simulink model "TxSteering_RxMVDR_4x4_HDL_IQ"  (R2021b)
settings: Solver=FixedStepDiscrete  StartTime=0.0  StopTime=stoptime  RelTol=1e-3
PreLoadFcn:
  | model_init
InitFcn:
  | model_init
model workspace (MAT data in the model file):
  socvcb : containers.Map (value not decoded)
values from neighbouring files (symbols this model uses):
  fc = ConverterSampleRate/4    (= 491520000)    [model_init.m]
  FPGAClkRate = DataSampleRate/VectorSamplingFactor    (= 245760000)    [model_init.m]
  movavg_bitshift = nextpow2(sqrt(windowSize))    [model_init.m]
  mvdrPipelineDelay = covMatDelay+movAvgDelay+matrixDivDelay+normResponseDelay    [model_init.m]
  NCO_bits = 14    [model_init.m]
  numArrayElements = 4    [model_init.m]
  S2MM_frame_size = testSrc1.FrameLength*testSrc1.SamplesPerSymbol*3    [model_init.m]
  testSrc1 = struct()    [model_init.m]
  testSrc2 = struct()    [model_init.m]
  windowSize = 4096    [model_init.m]
undefined symbols (not defined in the file or in its folder): j, physconst
libraries: hdlsllib x19, simulink x12, dspsrcs4 x2, embsystolicmatrixops x1, embreciprocals x1, dsphdlsigops x1, commrfcorlib x1
(part 2 of 3)

== system TxSteering_RxMVDR_4x4_HDL_IQ/DUT/Rx Data Capture/Stream FIFO  ==
  dataIn : Inport
  validIn : Inport  Port=2
  readyIn : Inport  Port=3
  Display : Display
  Logical Operator4 : Logic  Operator=NOT  IconShape=distinctive  AllPortsSameDT=off  OutDataTypeStr=boolean
  Logical Operator5 : Logic  IconShape=distinctive  AllPortsSameDT=off  OutDataTypeStr=boolean
  Logical Operator6 : Logic  Operator=NOT  IconShape=distinctive  AllPortsSameDT=off  OutDataTypeStr=boolean
  Logical Operator7 : Logic  IconShape=distinctive  AllPortsSameDT=off  OutDataTypeStr=boolean
  Signal Specification : SignalSpecification  SampleTime=1/FPGAClkRate
  Terminator : Terminator
  hdl_fwft_fifo : Subsystem  mask{FIFO_DEPTH=8192, AFULL_THRESH=4}
      mask prompts: FIFO_DEPTH "FIFO Depth"; AFULL_THRESH "Almost Full Threshold"
      mask init:
      | FIFO_CNT_BITS=ceil(log2(FIFO_DEPTH+1+3));
  dataOut : Outport  VectorParamsAs1DForOutWhenUnconnected=off
  ValidOut : Outport  Port=2  VectorParamsAs1DForOutWhenUnconnected=off
  readyOut : Outport  Port=3  VectorParamsAs1DForOutWhenUnconnected=off
  wires:
  Logical Operator4/1 -> Logical Operator5/2
  Logical Operator7/1 -> hdl_fwft_fifo/2(push)
  readyIn/1 -> Logical Operator5/1
  validIn/1 -> Logical Operator7/2
  hdl_fwft_fifo/2(empty) -> Logical Operator4/1
  hdl_fwft_fifo/3(num) -> Display/1
  dataIn/1 -> Signal Specification/1
  hdl_fwft_fifo/1(data_o) -> dataOut/1
  Logical Operator5/1 -> hdl_fwft_fifo/3(rd_ack), ValidOut/1
  Signal Specification/1 -> hdl_fwft_fifo/1(data_i)
  hdl_fwft_fifo/4(full) -> Terminator/1
  Logical Operator6/1 -> readyOut/1, Logical Operator7/1
  hdl_fwft_fifo/5(afull) -> Logical Operator6/1

== system TxSteering_RxMVDR_4x4_HDL_IQ/DUT/Rx Input Preparation/Apply Calibration Coefficients ==
  dataIn : Inport
  validIn : Inport  Port=2
  coeffIn : Inport  Port=3
  Data Type Duplicate : DataTypeDuplicate
  Data Type Conversion : DataTypeConversion
  Data Type Conversion1 : DataTypeConversion  OutDataTypeStr=input_dt  ConvertRealWorld=Stored Integer (SI)
  For Each Subsystem : Subsystem  TreatAsAtomicUnit=on
  Reshape : Reshape
  Reshape1 : Reshape  OutputDimensionality=Row vector (2-D)
  Reshape2 : Reshape
  Reshape3 : Reshape
  Selector : Selector  InputPortWidth=4  IndexOptions=Index vector (dialog)  Indices=1  OutputSizes=1
  dataOut : Outport
  validOut : Outport  Port=2
  wires:
  Data Type Conversion/1 -> Reshape1/1, Data Type Duplicate/2
  Reshape3/1 -> For Each Subsystem/3(coeffIn)
  Reshape2/1 -> For Each Subsystem/1(dataIn), Data Type Duplicate/1
  Reshape1/1 -> dataOut/1
  Reshape/1 -> Selector/1
  Selector/1 -> validOut/1
  For Each Subsystem/1(dataOut) -> Data Type Conversion/1
  For Each Subsystem/2(validOut) -> Reshape/1
  validIn/1 -> For Each Subsystem/2(validIn)
  dataIn/1 -> Data Type Conversion1/1
  coeffIn/1 -> Reshape3/1
  Data Type Conversion1/1 -> Reshape2/1

== system TxSteering_RxMVDR_4x4_HDL_IQ/DUT/Rx Input Preparation/From Data Bus ==
  bus : Inport
  Bus Selector : BusSelector  OutputSignals=data,valid
  data : Outport  VectorParamsAs1DForOutWhenUnconnected=off
  valid : Outport  Port=2  VectorParamsAs1DForOutWhenUnconnected=off
  wires:
  Bus Selector/2 -> valid/1  "<valid>"
  Bus Selector/1 -> data/1  "<data>"
  bus/1 -> Bus Selector/1

== system TxSteering_RxMVDR_4x4_HDL_IQ/DUT/Rx Input Preparation/To Data Bus ==
  data : Inport
  valid : Inport  Port=2
  Bus Creator : BusCreator  Inputs=2
  bus : Outport  VectorParamsAs1DForOutWhenUnconnected=off
  wires:
  valid/1 -> Bus Creator/2  "valid"
  data/1 -> Bus Creator/1  "data"
  Bus Creator/1 -> bus/1

== system TxSteering_RxMVDR_4x4_HDL_IQ/DUT/To DAC Interface/From Data Bus ==
  bus : Inport
  Bus Selector : BusSelector  OutputSignals=data,valid
  data : Outport  VectorParamsAs1DForOutWhenUnconnected=off
  valid : Outport  Port=2  VectorParamsAs1DForOutWhenUnconnected=off
  wires:
  Bus Selector/2 -> valid/1  "<valid>"
  Bus Selector/1 -> data/1  "<data>"
  bus/1 -> Bus Selector/1

== system TxSteering_RxMVDR_4x4_HDL_IQ/DUT/Tx Signal Generation/Calibration NCO ==
  inc : Inport
  Constant : Constant  Value=true  SampleTime=-1
  Data Type Conversion : DataTypeConversion  OutDataTypeStr=input_dt
  Mux : Mux
  NCO HDL Optimized : dsphdlsigops/NCO HDL Optimized  PhaseIncrementSource=Input port  PhaseIncrement=100  PhaseOffsetSource=Property  PhaseOffset=0  DitherSource=Property  NumDitherBits=4  SamplesPerFrame=1  LUTCompress=off  ResetAction=off  Waveform=Complex exponential  PhasePort=off  SimulateUsing=Code generation  AccumulatorWL=NCO_bits  PhaseQuantization=on  NumQuantizerAccumulatorBits=12  OutputDataType=Binary point scaling  OutputWL=NCO_bits  OutputFL=NCO_bits-1
      settings: SourceProductName=DSP System Toolbox HDL Support
  dataOut : Outport
  validOut : Outport  Port=2
  wires:
  inc/1 -> NCO HDL Optimized/1
  NCO HDL Optimized/2 -> validOut/1
  Constant/1 -> NCO HDL Optimized/2
  NCO HDL Optimized/1 -> Data Type Conversion/1
  Data Type Conversion/1 -> Mux/1, Mux/2, Mux/3, Mux/4
  Mux/1 -> dataOut/1

== system TxSteering_RxMVDR_4x4_HDL_IQ/DUT/Tx Signal Generation/Combine Channels ==
  dataIn : Inport
  validIn : Inport  Port=2
  Add : Sum
  Bit Shift : hdlsllib/Logic and Bit Operations/Bit Shift  mode=Shift Right Arithmetic  N=1
  Data Type Conversion : DataTypeConversion  OutDataTypeStr=int16
  Data Type Conversion1 : DataTypeConversion  OutDataTypeStr=input_dt  ConvertRealWorld=Stored Integer (SI)
  Delay{,1..4} (5 alike) : Delay  DelayLength=1
  Selector : Selector  InputPortWidth=2  IndexOptions=Index vector (dialog)  Indices=1  OutputSizes=1
  Selector1 : Selector  InputPortWidth=8  IndexOptions=Index vector (dialog)  Indices=1:4  OutputSizes=1
  Selector2 : Selector  InputPortWidth=8  IndexOptions=Index vector (dialog)  Indices=5:8  OutputSizes=1
  dataOut : Outport
  validOut : Outport  Port=2
  wires:
  Bit Shift/1 -> Data Type Conversion/1
  dataIn/1 -> Selector2/1, Selector1/1
  validIn/1 -> Selector/1
  Selector/1 -> Delay3/1
  Selector2/1 -> Delay1/1
  Selector1/1 -> Delay/1
  Delay/1 -> Add/1
  Delay1/1 -> Add/2
  Delay2/1 -> Bit Shift/1
  Add/1 -> Delay2/1
  Delay3/1 -> Delay4/1
  Delay4/1 -> validOut/1
  Data Type Conversion/1 -> Data Type Conversion1/1
  Data Type Conversion1/1 -> dataOut/1

== system TxSteering_RxMVDR_4x4_HDL_IQ/DUT/Tx Signal Generation/Generate Steering Channels ==
  dataIn : Inport  Partition=on  PartitionDimension=1  PartitionWidth=1  PartitionOffset=0
  validIn : Inport  Port=2
  gain : Inport  Port=3  Partition=on  PartitionDimension=1  PartitionWidth=1  PartitionOffset=0
  steeringCoeffs : Inport  Port=4  Partition=on  PartitionDimension=1  PartitionWidth=4  PartitionOffset=0
  Apply Gain : Subsystem
  Apply Steering Coefficients : Subsystem  TreatAsAtomicUnit=on
  Data Type Conversion : DataTypeConversion  OutDataTypeStr=fixdt(1,16,0)
  For Each : ForEach  DisableCoverage=on
  Selector : Selector  InputPortWidth=4  IndexOptions=Index vector (dialog)  Indices=1  OutputSizes=1
  dataOut : Outport  ConcatenationDimension=1
  validOut : Outport  Port=2  ConcatenationDimension=1
  wires:
  Data Type Conversion/1 -> dataOut/1
  Selector/1 -> validOut/1
  steeringCoeffs/1 -> Apply Steering Coefficients/3(coeffIn)
  Apply Steering Coefficients/1(dataOut) -> Data Type Conversion/1
  Apply Steering Coefficients/2(validOut) -> Selector/1
  Apply Gain/1(dataOut) -> Apply Steering Coefficients/1(dataIn)
  gain/1 -> Apply Gain/3(gain)
  Apply Gain/2(validOut) -> Apply Steering Coefficients/2(validIn)
  dataIn/1 -> Apply Gain/1(dataIn)
  validIn/1 -> Apply Gain/2(validIn)

== system TxSteering_RxMVDR_4x4_HDL_IQ/DUT/Tx Signal Generation/To Data Bus ==
  data : Inport
  valid : Inport  Port=2
  Bus Creator : BusCreator  Inputs=2
  bus : Outport  VectorParamsAs1DForOutWhenUnconnected=off
  wires:
  Bus Creator/1 -> bus/1
  data/1 -> Bus Creator/1  "data"
  valid/1 -> Bus Creator/2  "valid"

== system TxSteering_RxMVDR_4x4_HDL_IQ/DUT/Tx Signal Generation/To Data Bus1 ==
  data : Inport
  valid : Inport  Port=2
  Bus Creator : BusCreator  Inputs=2
  bus : Outport  VectorParamsAs1DForOutWhenUnconnected=off
  wires:
  valid/1 -> Bus Creator/2  "valid"
  data/1 -> Bus Creator/1  "data"
  Bus Creator/1 -> bus/1

== system TxSteering_RxMVDR_4x4_HDL_IQ/DUT/Tx Signal Generation/Tx Source LUT ==
  Constant : Constant  Value=true  SampleTime=-1
  Delay : Delay  DelayLength=1
  HDL Counter : hdlsllib/Sources/HDL Counter  CountType=Count limited  CountInit=0  CountStep=1  CountMax=length(testSrc1.Data)-1  CountFromType=Initial value  CountFrom=0  CountResetPort=off  CountLoadPort=off  CountEnbPort=off  CountDirPort=off  CountHitOutputPort=off  CountDataType=Unsigned  CountWordLen=nextpow2(length(testSrc1.Data))  CountFracLen=0  CountSampTime=1/FPGAClkRate
  HDL Counter1 : hdlsllib/Sources/HDL Counter  CountType=Count limited  CountInit=0  CountStep=1  CountMax=length(testSrc2.Data)-1  CountFromType=Initial value  CountFrom=0  CountResetPort=off  CountLoadPort=off  CountEnbPort=off  CountDirPort=off  CountHitOutputPort=off  CountDataType=Unsigned  CountWordLen=nextpow2(length(testSrc2.Data))  CountFracLen=0  CountSampTime=1/FPGAClkRate
  HW Delay : UnitDelay  SampleTime=-1  HasFrameUpgradeWarning=on
  HW Delay1 : UnitDelay  SampleTime=-1  HasFrameUpgradeWarning=on
  Mux : Mux  Inputs=2
  Source 1 LUT : LookupNDDirect  NumberOfTableDimensions=1  Table=testSrc1.Data  DiagnosticForOutOfRangeInput=Error  TableDataTypeStr=fixdt(1,16,15)
  Source 2 LUT : LookupNDDirect  NumberOfTableDimensions=1  Table=testSrc2.Data  DiagnosticForOutOfRangeInput=Error  TableDataTypeStr=fixdt(1,16,15)
  dataOut : Outport
  validOut : Outport  Port=2
  wires:
  Source 1 LUT/1 -> HW Delay/1
  HDL Counter/1 -> Source 1 LUT/1
  Source 2 LUT/1 -> HW Delay1/1
  HW Delay/1 -> Mux/1
  HW Delay1/1 -> Mux/2
  Mux/1 -> dataOut/1
  Constant/1 -> Delay/1
  Delay/1 -> validOut/1
  HDL Counter1/1 -> Source 2 LUT/1

== system TxSteering_RxMVDR_4x4_HDL_IQ/S2MM DMA Plant/Unpack to uint32/Enabled Subsystem ==
  dataIn : Inport
  Enable : EnablePort
  Extract Bits : simulink/Logic and Bit Operations/Extract Bits  bitsToExtract=Range of bits  numBits=8  bitIdxRange=[0 31]  outScalingMode=Treat bit field as an integer
  Extract Bits1 : simulink/Logic and Bit Operations/Extract Bits  bitsToExtract=Range of bits  numBits=8  bitIdxRange=[32 63]  outScalingMode=Treat bit field as an integer
  Extract Bits2 : simulink/Logic and Bit Operations/Extract Bits  bitsToExtract=Range of bits  numBits=8  bitIdxRange=[64 95]  outScalingMode=Treat bit field as an integer
  Extract Bits3 : simulink/Logic and Bit Operations/Extract Bits  bitsToExtract=Range of bits  numBits=8  bitIdxRange=[96 127]  outScalingMode=Treat bit field as an integer
  Matrix Concatenate : Concatenate  NumInputs=4  Mode=Multidimensional array
  Reshape : Reshape  OutputDimensionality=Row vector (2-D)
  Reshape1 : Reshape
  dataOut : Outport
  wires:
  dataIn/1 -> Reshape/1
  Extract Bits/1 -> Matrix Concatenate/1
  Extract Bits3/1 -> Matrix Concatenate/4
  Extract Bits2/1 -> Matrix Concatenate/3
  Extract Bits1/1 -> Matrix Concatenate/2
  Reshape/1 -> Extract Bits/1, Extract Bits1/1, Extract Bits2/1, Extract Bits3/1
  Matrix Concatenate/1 -> Reshape1/1
  Reshape1/1 -> dataOut/1

== system TxSteering_RxMVDR_4x4_HDL_IQ/DUT/Rx Beamforming/Input Gate/From Data Bus ==
  bus : Inport
  Bus Selector : BusSelector  OutputSignals=data,valid
  data : Outport  VectorParamsAs1DForOutWhenUnconnected=off
  valid : Outport  Port=2  VectorParamsAs1DForOutWhenUnconnected=off
  wires:
  Bus Selector/2 -> valid/1  "<valid>"
  Bus Selector/1 -> data/1  "<data>"
  bus/1 -> Bus Selector/1

== system TxSteering_RxMVDR_4x4_HDL_IQ/DUT/Rx Beamforming/Input Gate/To Data Bus ==
  data : Inport
  valid : Inport  Port=2
  Bus Creator : BusCreator  Inputs=2
  bus : Outport  VectorParamsAs1DForOutWhenUnconnected=off
  wires:
  valid/1 -> Bus Creator/2  "valid"
  data/1 -> Bus Creator/1  "data"
  Bus Creator/1 -> bus/1

== system TxSteering_RxMVDR_4x4_HDL_IQ/DUT/Rx Beamforming/Input Gate/To Data Bus1 ==
  data : Inport
  valid : Inport  Port=2
  Bus Creator : BusCreator  Inputs=2
  bus : Outport  VectorParamsAs1DForOutWhenUnconnected=off
  wires:
  Bus Creator/1 -> bus/1
  data/1 -> Bus Creator/1  "data"
  valid/1 -> Bus Creator/2  "valid"

== system TxSteering_RxMVDR_4x4_HDL_IQ/DUT/Rx Beamforming/MVDR/Compute Weight Vector ==
  covarianceMatrix : Inport
  validIn : Inport  Port=2
  steeringVector : Inport  Port=3
  Complex Partial-Systolic Matrix Solve Using QR Decomposition : embsystolicmatrixops/Complex Partial-Systolic Matrix Solve Using QR Decomposition  m=4  n=4  p=1  regularizationParameter=0  OutputType=fixdt(1,32,15)
      settings: SourceProductBaseCode=SL
  Constant : Constant  Value=false  SampleTime=-1
  Data Type Conversion1 : DataTypeConversion  OutDataTypeStr=matrixdivin_dt
  Data Type Conversion2 : DataTypeConversion  OutDataTypeStr=matrixdivin_dt
  Data Type Conversion4 : DataTypeConversion  OutDataTypeStr=matrixdivout_dt
  Deserialize Output Data : Subsystem
  Reshape1 : Reshape  OutputDimensionality=Column vector (2-D)  OutputDimensions=[4,4]
  Serialize Input Data : Subsystem
  w : Outport
  validOut : Outport  Port=2
  wires:
  covarianceMatrix/1 -> Data Type Conversion1/1
  steeringVector/1 -> Data Type Conversion2/1
  Data Type Conversion2/1 -> Reshape1/1
  validIn/1 -> Serialize Input Data/3(validIn)
  Constant/1 -> Complex Partial-Systolic Matrix Solve Using QR Decomposition/4
  Serialize Input Data/3(validOut) -> Complex Partial-Systolic Matrix Solve Using QR Decomposition/3  "validIn"
  Complex Partial-Systolic Matrix Solve Using QR Decomposition/3 -> Serialize Input Data/4(readyIn)
  Serialize Input Data/1(AOut) -> Complex Partial-Systolic Matrix Solve Using QR Decomposition/1
  Reshape1/1 -> Serialize Input Data/2(BIn)
  Complex Partial-Systolic Matrix Solve Using QR Decomposition/1 -> Data Type Conversion4/1
  Data Type Conversion4/1 -> Deserialize Output Data/1(dataIn)
  Complex Partial-Systolic Matrix Solve Using QR Decomposition/2 -> Deserialize Output Data/2(validIn)
  Deserialize Output Data/1(dataOut) -> w/1
  Deserialize Output Data/2(validOut) -> validOut/1
  Serialize Input Data/2(BOut) -> Complex Partial-Systolic Matrix Solve Using QR Decomposition/2
  Data Type Conversion1/1 -> Serialize Input Data/1(AIn)

== system TxSteering_RxMVDR_4x4_HDL_IQ/DUT/Rx Beamforming/MVDR/Form Beam ==
  Bus Element In : Inport  PortName=dataBusIn  Element=data
  Bus Element In1 : Inport  PortName=dataBusIn  Element=valid
  w : Inport  Port=2
  Data Type Conversion : DataTypeConversion  OutDataTypeStr=output_dt
  Delay1 : Delay  DelayLength=6
  Delay2 : Delay
  Delay3 : Delay  DelayLength=mvdrPipelineDelay
  Delay5 : Delay  DelayLength=mvdrPipelineDelay
  Math Function2 : Math  Operator=conj  SaturateOnIntegerOverflow=on
  Parallel Complex Multiply : Subsystem  TreatAsAtomicUnit=on
  Reshape : Reshape
  Reshape1 : Reshape
  Rx Beam - Spectrum : SpectrumAnalyzer
  Tree Sum : Subsystem
  Bus Element Out : Outport  PortName=dataBusOut  Element=data
  Out Bus Element : Outport  PortName=dataBusOut  Element=valid
  wires:
  Bus Element In/1 -> Delay5/1
  Parallel Complex Multiply/1(z) -> Tree Sum/1(In1)
  Tree Sum/1(Out1) -> Data Type Conversion/1
  Math Function2/1 -> Reshape/1
  w/1 -> Math Function2/1
  Reshape/1 -> Parallel Complex Multiply/2(z2)
  Reshape1/1 -> Parallel Complex Multiply/1(z1)
  Data Type Conversion/1 -> Rx Beam - Spectrum/1, Bus Element Out/1
  Delay2/1 -> Out Bus Element/1
  Delay1/1 -> Delay2/1
  Bus Element In1/1 -> Delay3/1
  Delay5/1 -> Reshape1/1
  Delay3/1 -> Delay1/1

== system TxSteering_RxMVDR_4x4_HDL_IQ/DUT/Rx Beamforming/MVDR/Form Covariance Matrix ==
  Bus Element In : Inport  PortName=dataBusIn  Element=data
  Bus Element In1 : Inport  PortName=dataBusIn  Element=valid
  Conj : Math  Operator=conj
  Data Type Conversion : DataTypeConversion  OutDataTypeStr=covmat_dt
  Data Type Conversion1 : DataTypeConversion  OutDataTypeStr=adc_dt
  Delay : Delay  DelayLength=6
  Matrix Multiply Partitioned : Subsystem  TreatAsAtomicUnit=on
  Reshape : Reshape
  dataOut : Outport
  validOut : Outport  Port=2
  wires:
  Bus Element In1/1 -> Delay/1
  Bus Element In/1 -> Data Type Conversion1/1
  Reshape/1 -> Conj/1, Matrix Multiply Partitioned/1(x)  "x"
  Matrix Multiply Partitioned/1(C) -> Data Type Conversion/1  "x * x'"
  Delay/1 -> validOut/1
  Conj/1 -> Matrix Multiply Partitioned/2(x_conj)
  Data Type Conversion1/1 -> Reshape/1
  Data Type Conversion/1 -> dataOut/1

== system TxSteering_RxMVDR_4x4_HDL_IQ/DUT/Rx Beamforming/MVDR/Moving Average ==
  note: Shift replaces gain by 1/sqrt(windowSize)
  dataIn : Inport
  validIn : Inport  Port=2
  Add : Sum  Inputs=++-  AccumDataTypeStr=movavg_accum_dt  OutDataTypeStr=Inherit: Same as accumulator
  Bit Shift : hdlsllib/Logic and Bit Operations/Bit Shift  mode=Shift Right Arithmetic  N=movavg_bitshift
  Data Type Conversion : DataTypeConversion  OutDataTypeStr=movavg_out_dt
  Delay : Delay  DelayLength=windowSize
  Delay{1..5} (5 alike) : Delay  DelayLength=1
  Reshape : Reshape  OutputDimensionality=Customize  OutputDimensions=[4,4]
  Reshape1 : Reshape  OutputDimensions=[4,4]
  Wait for Running Sum Init : Subsystem
  dataOut : Outport
  validOut : Outport  Port=2
  wires:
  Bit Shift/1 -> Data Type Conversion/1
  Delay1/1 -> Bit Shift/1, Add/1
  Delay/1 -> Add/3
  Add/1 -> Delay1/1
  dataIn/1 -> Delay2/1
  validIn/1 -> Delay3/1
  Delay2/1 -> Reshape1/1
  Delay4/1 -> dataOut/1
  Delay5/1 -> validOut/1
  Delay3/1 -> Wait for Running Sum Init/1(In1)
  Wait for Running Sum Init/1(Out1) -> Delay5/1
  Data Type Conversion/1 -> Reshape/1
  Reshape/1 -> Delay4/1
  Reshape1/1 -> Delay/1, Add/2

== system TxSteering_RxMVDR_4x4_HDL_IQ/DUT/Rx Beamforming/MVDR/Normalize Response ==
  note: This subsystem scales the weight vector to ensure unit gain in the target direction.
  wIn : Inport
  validIn : Inport  Port=2
  steeringVector : Inport  Port=3
  MVDR Weight Update : Subsystem
  Unit Delay Enabled Synchronous : hdlsllib/Discrete/Unit Delay Enabled Synchronous  InitialCondition=0.0  SampleTime=-1
      settings: SourceProductBaseCode=SL
  wOut : Outport
  wires:
  steeringVector/1 -> MVDR Weight Update/1(Steering Vector)
  wIn/1 -> MVDR Weight Update/2(x)
  MVDR Weight Update/1(w) -> Unit Delay Enabled Synchronous/1
  MVDR Weight Update/2(validOut) -> Unit Delay Enabled Synchronous/2
  Unit Delay Enabled Synchronous/1 -> wOut/1
  validIn/1 -> MVDR Weight Update/3(validIn)

== system TxSteering_RxMVDR_4x4_HDL_IQ/DUT/Rx Beamforming/Output Selector/RepackageInput ==
  In1 : Inport
  Bus Creator : BusCreator  Inputs=2
  Bus Selector : BusSelector  OutputSignals=data,valid
  Pack Complex Vector : Subsystem  mask(Pack Complex Vector){}
      mask help:
      | Convert complex vector to packed word.
      |
      | Real and imaginary components are interleaved, with real component starting in LSB position.
      |
      | The first vector element is placed in the LSB, and the last vector element is placed in the MSB.
      mask Display: fprintf('Pack\nComplex\nVector');
  Out1 : Outport
  wires:
  In1/1 -> Bus Selector/1
  Bus Creator/1 -> Out1/1
  Bus Selector/2 -> Bus Creator/2  "<valid>"
  Bus Selector/1 -> Pack Complex Vector/1(u)  "<data>"
  Pack Complex Vector/1(y) -> Bus Creator/1  "data"

== system TxSteering_RxMVDR_4x4_HDL_IQ/DUT/Rx Beamforming/Output Selector/RepackageMVDR ==
  In3 : Inport
  Bus Creator : BusCreator  Inputs=2
  Bus Selector : BusSelector  OutputSignals=data,valid
  Data Type Conversion1 : DataTypeConversion  OutDataTypeStr=fixdt(0,128,0)
  Pack Complex : Subsystem  mask(Pack Complex){dummy=0}
      mask help:
      | Convert complex value to packed word.
      |
      | Real component goes to lower bits; imaginary component goes to upper bits.
      mask Display: fprintf('Pack\nComplex');
  Out1 : Outport
  wires:
  Pack Complex/1(Out1) -> Data Type Conversion1/1
  Data Type Conversion1/1 -> Bus Creator/1  "data"
  Bus Selector/2 -> Bus Creator/2  "<valid>"
  In3/1 -> Bus Selector/1
  Bus Creator/1 -> Out1/1
  Bus Selector/1 -> Pack Complex/1(In1)  "<data>"

== system TxSteering_RxMVDR_4x4_HDL_IQ/DUT/Rx Data Capture/CaptureTriggerControl/AXI4-Lite Initial Value ==
  In1 : Inport
  Compare To Zero : simulink/Logic and Bit Operations/Compare To Zero  relop=~=  OutDataTypeStr=boolean
  Logical Operator : Logic  Operator=OR  IconShape=distinctive  AllPortsSameDT=off  OutDataTypeStr=boolean
  Set_Latch : Subsystem
  Unit Delay Enabled Synchronous : hdlsllib/Discrete/Unit Delay Enabled Synchronous  InitialCondition=x0  SampleTime=-1
      settings: SourceProductBaseCode=SL
  Out1 : Outport  VectorParamsAs1DForOutWhenUnconnected=off
  wires:
  In1/1 -> Unit Delay Enabled Synchronous/1, Compare To Zero/1
  Logical Operator/1 -> Unit Delay Enabled Synchronous/2
  Compare To Zero/1 -> Logical Operator/1, Set_Latch/1(S)
  Set_Latch/1(Q) -> Logical Operator/2
  Unit Delay Enabled Synchronous/1 -> Out1/1

== system TxSteering_RxMVDR_4x4_HDL_IQ/DUT/Rx Data Capture/CaptureTriggerControl/AutoTrigger ==
  MaxCount : Inport
  En : Inport  Port=2
  DataPushFrequency : hdlsllib/Sources/HDL Counter  CountType=Free running  CountInit=0  CountStep=1  CountMax=25  CountFromType=Initial value  CountFrom=0  CountResetPort=on  CountLoadPort=off  CountEnbPort=on  CountDirPort=off  CountHitOutputPort=off  CountDataType=Unsigned  CountWordLen=32  CountFracLen=0  CountSampTime=1
  Relational Operator : RelationalOperator  Operator===  OutDataTypeStr=boolean  RndMeth=Simplest
  Trig : Outport  VectorParamsAs1DForOutWhenUnconnected=off
  wires:
  DataPushFrequency/1 -> Relational Operator/2
  Relational Operator/1 -> Trig/1, DataPushFrequency/1
  En/1 -> DataPushFrequency/2
  MaxCount/1 -> Relational Operator/1

== system TxSteering_RxMVDR_4x4_HDL_IQ/DUT/Rx Data Capture/FIFOControl/HandleDefaultValue ==
  In1 : Inport
  Compare To Zero1 : simulink/Logic and Bit Operations/Compare To Zero  relop=~=  OutDataTypeStr=boolean
  Constant : Constant  Value=1024  OutDataTypeStr=uint32  SampleTime=-1
  Switch : Switch  Criteria=u2 ~= 0
  Out1 : Outport
  wires:
  Compare To Zero1/1 -> Switch/2
  Constant/1 -> Switch/3
  Switch/1 -> Out1/1
  In1/1 -> Compare To Zero1/1, Switch/1

== system TxSteering_RxMVDR_4x4_HDL_IQ/DUT/Rx Data Capture/FIFOControl/sr_latch ==
  S : Inport
  R : Inport  Port=2
  Logical Operator1 : Logic  IconShape=distinctive  AllPortsSameDT=off  OutDataTypeStr=boolean
  Logical Operator2 : Logic  Operator=NOT  IconShape=distinctive  AllPortsSameDT=off  OutDataTypeStr=boolean
  Logical Operator9 : Logic  Operator=OR  IconShape=distinctive  AllPortsSameDT=off  OutDataTypeStr=boolean
  Unit Delay1 : UnitDelay  SampleTime=-1  HasFrameUpgradeWarning=on
  Q : Outport  VectorParamsAs1DForOutWhenUnconnected=off
  wires:
  S/1 -> Logical Operator9/1
  R/1 -> Logical Operator2/1
  Logical Operator2/1 -> Logical Operator1/1
  Unit Delay1/1 -> Logical Operator1/2, Q/1
  Logical Operator9/1 -> Unit Delay1/1
  Logical Operator1/1 -> Logical Operator9/2

== system TxSteering_RxMVDR_4x4_HDL_IQ/DUT/Rx Data Capture/Stream FIFO /hdl_fwft_fifo ==
  data_i : Inport
  push : Inport  Port=2
  rd_ack : Inport  Port=3
  Compare To Constant : simulink/Logic and Bit Operations/Compare To Constant  relop=>=  const=FIFO_DEPTH-AFULL_THRESH  OutDataTypeStr=boolean
  HDL FIFO : hdlsllib/HDL RAMs/HDL FIFO  fifo_size=FIFO_DEPTH  mode=FWFT  ratio=1  push_msg=Error  pop_msg=Ignore  show_empty=on  show_full=on  show_num=on  LabelModeActiveChoice_Mode=FWFT
      settings: SourceProductBaseCode=SL
  Logical Operator1 : Logic  Operator=NOT  IconShape=distinctive  AllPortsSameDT=off  OutDataTypeStr=boolean
  Logical Operator2 : Logic  IconShape=distinctive  AllPortsSameDT=off  OutDataTypeStr=boolean
  data_o : Outport  VectorParamsAs1DForOutWhenUnconnected=off
  empty : Outport  Port=2  VectorParamsAs1DForOutWhenUnconnected=off
  num : Outport  Port=3  VectorParamsAs1DForOutWhenUnconnected=off
  full : Outport  Port=4  VectorParamsAs1DForOutWhenUnconnected=off
  afull : Outport  Port=5  VectorParamsAs1DForOutWhenUnconnected=off
  wires:
  Compare To Constant/1 -> afull/1
  data_i/1 -> HDL FIFO/1
  push/1 -> Logical Operator2/1
  Logical Operator2/1 -> HDL FIFO/2
  Logical Operator1/1 -> Logical Operator2/2
  HDL FIFO/3 -> Logical Operator1/1, full/1
  HDL FIFO/4 -> Compare To Constant/1, num/1
  HDL FIFO/2 -> empty/1
  HDL FIFO/1 -> data_o/1
  rd_ack/1 -> HDL FIFO/3

== system TxSteering_RxMVDR_4x4_HDL_IQ/DUT/Rx Input Preparation/Apply Calibration Coefficients/For Each Subsystem ==
  dataIn : Inport  Partition=on  PartitionDimension=1  PartitionWidth=1  PartitionOffset=0
  validIn : Inport  Port=2
  coeffIn : Inport  Port=3  Partition=on  PartitionDimension=1  PartitionWidth=1  PartitionOffset=0
  For Each : ForEach  DisableCoverage=on
  HDL Complex Multiplier : Subsystem
  dataOut : Outport  ConcatenationDimension=1
  validOut : Outport  Port=2  ConcatenationDimension=1
  wires:
  HDL Complex Multiplier/2(validOut) -> validOut/1
  HDL Complex Multiplier/1(z) -> dataOut/1
  validIn/1 -> HDL Complex Multiplier/3(validIn)
  coeffIn/1 -> HDL Complex Multiplier/2(z2)
  dataIn/1 -> HDL Complex Multiplier/1(z1)

== system TxSteering_RxMVDR_4x4_HDL_IQ/DUT/Tx Signal Generation/Generate Steering Channels/Apply Gain ==
  dataIn : Inport
  validIn : Inport  Port=2
  gain : Inport  Port=3
  Data Type Duplicate : DataTypeDuplicate
  Data Type Conversion1 : DataTypeConversion
  Data Type Conversion2 : DataTypeConversion  OutDataTypeStr=int16  ConvertRealWorld=Stored Integer (SI)  LockScale=on
  PipelineDelay : Delay
  PipelineDelay1 : Delay
  PipelineDelay2 : Delay  DelayLength=1
  PipelineDelay3 : Delay
  PipelineDelay4 : Delay  DelayLength=1
  Product : Product
  dataOut : Outport
  validOut : Outport  Port=2  VectorParamsAs1DForOutWhenUnconnected=off
  wires:
  dataIn/1 -> Data Type Conversion2/1
  gain/1 -> PipelineDelay/1
  PipelineDelay/1 -> Product/1
  PipelineDelay1/1 -> Product/2
  Product/1 -> PipelineDelay2/1
  PipelineDelay2/1 -> Data Type Conversion1/1
  Data Type Conversion1/1 -> dataOut/1, Data Type Duplicate/2
  Data Type Conversion2/1 -> Data Type Duplicate/1, PipelineDelay1/1
  validIn/1 -> PipelineDelay3/1
  PipelineDelay3/1 -> PipelineDelay4/1
  PipelineDelay4/1 -> validOut/1

== system TxSteering_RxMVDR_4x4_HDL_IQ/DUT/Tx Signal Generation/Generate Steering Channels/Apply Steering Coefficients ==
  dataIn : Inport
  validIn : Inport  Port=2
  coeffIn : Inport  Port=3  Partition=on  PartitionDimension=1  PartitionWidth=1  PartitionOffset=0
  For Each : ForEach  DisableCoverage=on
  HDL Complex Multiplier : Subsystem
  dataOut : Outport  ConcatenationDimension=1
  validOut : Outport  Port=2  ConcatenationDimension=1
  wires:
  dataIn/1 -> HDL Complex Multiplier/1(z1)
  coeffIn/1 -> HDL Complex Multiplier/2(z2)
  validIn/1 -> HDL Complex Multiplier/3(validIn)
  HDL Complex Multiplier/1(z) -> dataOut/1
  HDL Complex Multiplier/2(validOut) -> validOut/1

== system TxSteering_RxMVDR_4x4_HDL_IQ/DUT/Rx Beamforming/MVDR/Compute Weight Vector/Deserialize Output Data ==
  dataIn : Inport
  validIn : Inport  Port=2
  AND : Logic  IconShape=distinctive  AllPortsSameDT=off  OutDataTypeStr=boolean
  Assignment : Assignment  IndexMode=Zero-based  DiagnosticForDimensions=Warning  IndexOptions=Index vector (port)  Indices=1  OutputSizes=4
  Compare To Constant : simulink/Logic and Bit Operations/Compare To Constant  relop===  const=3.0  OutDataTypeStr=boolean
  Data Type Duplicate : DataTypeDuplicate
  Data Type Conversion : DataTypeConversion  OutDataTypeStr=uint8
  Delay : Delay  DelayLength=1
  Delay1 : Delay  DelayLength=1
  HDL Counter : hdlsllib/Sources/HDL Counter  CountType=Free running  CountInit=0  CountStep=1  CountMax=25  CountFromType=Initial value  CountFrom=0  CountResetPort=off  CountLoadPort=off  CountEnbPort=on  CountDirPort=off  CountHitOutputPort=off  CountDataType=Unsigned  CountWordLen=2  CountFracLen=0  CountSampTime=1
  Unit Delay Enabled Synchronous : hdlsllib/Discrete/Unit Delay Enabled Synchronous  InitialCondition=complex(zeros(4,1))  SampleTime=-1
      settings: SourceProductBaseCode=SL
  Unit Delay Enabled Synchronous1 : hdlsllib/Discrete/Unit Delay Enabled Synchronous  InitialCondition=0  SampleTime=-1
      settings: SourceProductBaseCode=SL
  dataOut : Outport
  validOut : Outport  Port=2
  wires:
  AND/1 -> Delay/1
  HDL Counter/1 -> Compare To Constant/1, Data Type Conversion/1
  dataIn/1 -> Data Type Duplicate/1, Assignment/2
  Compare To Constant/1 -> AND/1
  Delay/1 -> Delay1/1, Unit Delay Enabled Synchronous1/2
  Data Type Conversion/1 -> Assignment/3
  validIn/1 -> HDL Counter/1, Unit Delay Enabled Synchronous/2, AND/2
  Assignment/1 -> Unit Delay Enabled Synchronous/1
  Unit Delay Enabled Synchronous/1 -> Assignment/1, Data Type Duplicate/2, Unit Delay Enabled Synchronous1/1
  Delay1/1 -> validOut/1
  Unit Delay Enabled Synchronous1/1 -> dataOut/1

== system TxSteering_RxMVDR_4x4_HDL_IQ/DUT/Rx Beamforming/MVDR/Compute Weight Vector/Serialize Input Data ==
  AIn : Inport
  BIn : Inport  Port=2
  validIn : Inport  Port=3
  readyIn : Inport  Port=4
  AND : Logic  IconShape=distinctive  AllPortsSameDT=off  OutDataTypeStr=boolean
  Compare To Constant : simulink/Logic and Bit Operations/Compare To Constant  relop===  const=0  OutDataTypeStr=boolean
  Detect Rise Positive : simulink/Logic and Bit Operations/Detect Rise Positive  vinit=0  OutDataTypeStr=boolean
  HDL Counter : hdlsllib/Sources/HDL Counter  CountType=Free running  CountInit=0  CountStep=1  CountMax=25  CountFromType=Initial value  CountFrom=0  CountResetPort=off  CountLoadPort=off  CountEnbPort=on  CountDirPort=off  CountHitOutputPort=off  CountDataType=Unsigned  CountWordLen=2  CountFracLen=0  CountSampTime=1
  Output Selector : Subsystem
  Output Selector1 : Subsystem
  Unit Delay : UnitDelay  SampleTime=-1  HasFrameUpgradeWarning=on
  Unit Delay Enabled Synchronous1 : hdlsllib/Discrete/Unit Delay Enabled Synchronous  InitialCondition=0.0  SampleTime=-1
      settings: SourceProductBaseCode=SL
  Unit Delay Enabled Synchronous2 : hdlsllib/Discrete/Unit Delay Enabled Synchronous  InitialCondition=0.0  SampleTime=-1
      settings: SourceProductBaseCode=SL
  readyQueue : MATLAB Function  TreatAsAtomicUnit=on
  AOut : Outport
  BOut : Outport  Port=2
  validOut : Outport  Port=3
  wires:
  readyIn/1 -> Detect Rise Positive/1
  HDL Counter/1 -> Compare To Constant/1, Output Selector1/1(idx), Output Selector/1(idx)
  Compare To Constant/1 -> AND/1
  readyQueue/1(validOut) -> HDL Counter/1, AND/2, validOut/1
  Detect Rise Positive/1 -> readyQueue/1(readyEdge)
  AIn/1 -> Unit Delay Enabled Synchronous1/1
  validIn/1 -> Unit Delay Enabled Synchronous2/2, Unit Delay Enabled Synchronous1/2, Unit Delay/1
  Unit Delay/1 -> readyQueue/2(validIn)
  BIn/1 -> Unit Delay Enabled Synchronous2/1
  AND/1 -> Output Selector1/2(first), Output Selector/2(first)
  Unit Delay Enabled Synchronous1/1 -> Output Selector/3(dataIn)
  Output Selector/1(dataOut) -> AOut/1
  Unit Delay Enabled Synchronous2/1 -> Output Selector1/3(dataIn)
  Output Selector1/1(dataOut) -> BOut/1

== system TxSteering_RxMVDR_4x4_HDL_IQ/DUT/Rx Beamforming/MVDR/Form Beam/Parallel Complex Multiply ==
  z1 : Inport  Partition=on  PartitionDimension=1  PartitionWidth=1  PartitionOffset=0
  z2 : Inport  Port=2  Partition=on  PartitionDimension=1  PartitionWidth=1  PartitionOffset=0
  For Each : ForEach  DisableCoverage=on
  HDL Complex Multiply : Subsystem  mask(HDL Complex Multiplier (3 Multiply, 5 Add)){D1=2, D2=1, D3=1, D4=1, D5=1}
      mask help:
      | Xilinx devices:
      | - Set D1 = 1 or 2 to trade off speed & FF resources
      | - Set D2-D5 = 1 to fully leverage DSP48 pipelines
      | - Use sync reset
      |
      | Intel FPGAs:
      | - Set D1 = 1 or 2 depending on device family
      | - Set D5 = 1; D2, D3, D4 = 0
      | - Use async reset
      mask init:
      | delay = D1+D2+D3+D4+D5;
      mask Display:
      | fprintf('Delay=%d',delay);
      | port_label('input',1,'z1');
      | port_label('input',2,'z2');
  z : Outport  ConcatenationDimension=1
  wires:
  z1/1 -> HDL Complex Multiply/1(In1)
  z2/1 -> HDL Complex Multiply/2(In2)
  HDL Complex Multiply/1(Out1) -> z/1

== system TxSteering_RxMVDR_4x4_HDL_IQ/DUT/Rx Beamforming/MVDR/Form Beam/Tree Sum ==
  In1 : Inport
  Delay3 : Delay  DelayLength=ceil(log2(numArrayElements))
  Tree Sum of Elements : Sum  Inputs=+  OutDataTypeStr=Inherit: Same as first input  LockScale=on
  Out1 : Outport
  wires:
  Delay3/1 -> Out1/1
  In1/1 -> Tree Sum of Elements/1
  Tree Sum of Elements/1 -> Delay3/1

== system TxSteering_RxMVDR_4x4_HDL_IQ/DUT/Rx Beamforming/MVDR/Form Covariance Matrix/Matrix Multiply Partitioned ==
  x : Inport
  x_conj : Inport  Port=2
  Partition x_conj : Subsystem
  Reshape : Reshape  OutputDimensionality=Customize  OutputDimensions=[4,4]
  C : Outport
  wires:
  x/1 -> Partition x_conj/1(x)
  x_conj/1 -> Partition x_conj/2(x_conj)
  Partition x_conj/1(C) -> Reshape/1
  Reshape/1 -> C/1

== system TxSteering_RxMVDR_4x4_HDL_IQ/DUT/Rx Beamforming/MVDR/Moving Average/Wait for Running Sum Init ==
  In1 : Inport
  Compare To Constant : simulink/Logic and Bit Operations/Compare To Constant  relop=<  const=windowSize  OutDataTypeStr=boolean
  HDL Counter : hdlsllib/Sources/HDL Counter  CountType=Free running  CountInit=0  CountStep=1  CountMax=25  CountFromType=Initial value  CountFrom=0  CountResetPort=off  CountLoadPort=off  CountEnbPort=on  CountDirPort=off  CountHitOutputPort=off  CountDataType=Unsigned  CountWordLen=nextpow2(windowSize)+1  CountFracLen=0  CountSampTime=1
  Logical Operator : Logic  IconShape=distinctive  AllPortsSameDT=off  OutDataTypeStr=boolean
  Logical Operator1 : Logic  IconShape=distinctive  AllPortsSameDT=off  OutDataTypeStr=boolean
  Logical Operator2 : Logic  Operator=NOT  IconShape=distinctive  AllPortsSameDT=off  OutDataTypeStr=boolean
  Out1 : Outport
  wires:
  Logical Operator2/1 -> Logical Operator/2
  Logical Operator1/1 -> HDL Counter/1
  Compare To Constant/1 -> Logical Operator1/2, Logical Operator2/1
  Logical Operator/1 -> Out1/1
  HDL Counter/1 -> Compare To Constant/1
  In1/1 -> Logical Operator1/1, Logical Operator/1

== system TxSteering_RxMVDR_4x4_HDL_IQ/DUT/Rx Beamforming/MVDR/Normalize Response/MVDR Weight Update ==
  Steering Vector : Inport
  x : Inport  Port=2
  validIn : Inport  Port=3
  Delay{,1,3..6} (6 alike) : Delay  DelayLength=1
  Delay2 : Delay  DelayLength=8
  Inner Product : Subsystem
  Vector / Scalar Divide : Subsystem
  w : Outport
  validOut : Outport  Port=2
  wires:
  x/1 -> Delay3/1
  Vector / Scalar Divide/1(w) -> w/1
  Delay4/1 -> Inner Product/1(u)
  Inner Product/1(y) -> Delay5/1
  Delay6/1 -> Vector / Scalar Divide/1(x)
  Delay/1 -> Vector / Scalar Divide/3(validIn)
  Steering Vector/1 -> Delay4/1
  Delay3/1 -> Delay2/1, Inner Product/2(v)
  Delay5/1 -> Vector / Scalar Divide/2(y)
  Inner Product/2(validOut) -> Delay/1
  validIn/1 -> Delay1/1
  Vector / Scalar Divide/2(validOut) -> validOut/1
  Delay1/1 -> Inner Product/3(validIn)
  Delay2/1 -> Delay6/1

== system TxSteering_RxMVDR_4x4_HDL_IQ/DUT/Rx Beamforming/Output Selector/RepackageInput/Pack Complex Vector ==
  u : Inport
  pack_vector_complex : MATLAB Function  TreatAsAtomicUnit=on
  y : Outport
  wires:
  pack_vector_complex/1(y) -> y/1
  u/1 -> pack_vector_complex/1(u)

== system TxSteering_RxMVDR_4x4_HDL_IQ/DUT/Rx Beamforming/Output Selector/RepackageMVDR/Pack Complex ==
  In1 : Inport
  Bit Concat : hdlsllib/Logic and Bit Operations/Bit Concat  numInputs=2
  Complex to Real-Imag : ComplexToRealImag
  Out1 : Outport  VectorParamsAs1DForOutWhenUnconnected=off
  wires:
  Complex to Real-Imag/2 -> Bit Concat/1
  Complex to Real-Imag/1 -> Bit Concat/2
  Bit Concat/1 -> Out1/1
  In1/1 -> Complex to Real-Imag/1

== system TxSteering_RxMVDR_4x4_HDL_IQ/DUT/Rx Data Capture/CaptureTriggerControl/AXI4-Lite Initial Value/Set_Latch ==
  S : Inport
  Logical Operator5 : Logic  Operator=OR  IconShape=distinctive  AllPortsSameDT=off  OutDataTypeStr=boolean
  Unit Delay : UnitDelay  SampleTime=-1  HasFrameUpgradeWarning=on
  Q : Outport  VectorParamsAs1DForOutWhenUnconnected=off
  wires:
  Logical Operator5/1 -> Unit Delay/1
  S/1 -> Logical Operator5/1
  Unit Delay/1 -> Q/1, Logical Operator5/2

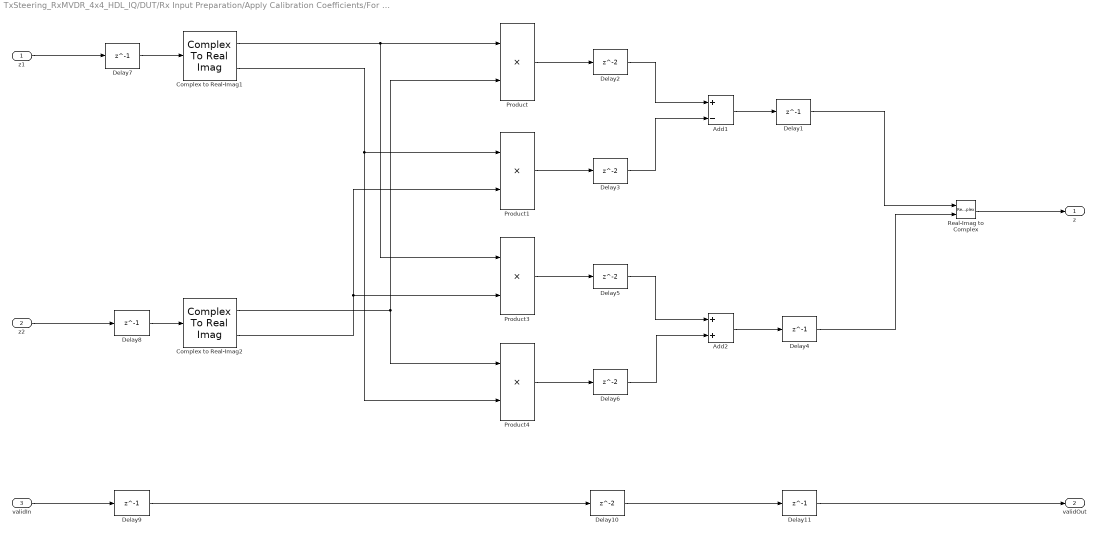
== system TxSteering_RxMVDR_4x4_HDL_IQ/DUT/Rx Input Preparation/Apply Calibration Coefficients/For Each Subsystem/HDL Complex Multiplier ==
  z1 : Inport
  z2 : Inport  Port=2
  validIn : Inport  Port=3
  Add1 : Sum  Inputs=+-
  Add2 : Sum
  Complex to Real-Imag1 : ComplexToRealImag
  Complex to Real-Imag2 : ComplexToRealImag
  Delay{1,4,7..9,11} (6 alike) : Delay  DelayLength=1  InitialCondition=0  InputProcessing=Columns as channels (frame based)
  Delay{2..3,5..6,10} (5 alike) : Delay  InitialCondition=0  InputProcessing=Columns as channels (frame based)
  Product{,1,3..4} (4 alike) : Product
  Real-Imag to Complex : RealImagToComplex
  z : Outport  VectorParamsAs1DForOutWhenUnconnected=off
  validOut : Outport  Port=2  VectorParamsAs1DForOutWhenUnconnected=off
  wires:
  Delay11/1 -> validOut/1
  Delay10/1 -> Delay11/1
  Delay9/1 -> Delay10/1
  validIn/1 -> Delay9/1
  Delay8/1 -> Complex to Real-Imag2/1
  Delay7/1 -> Complex to Real-Imag1/1
  Delay4/1 -> Real-Imag to Complex/2
  Delay1/1 -> Real-Imag to Complex/1
  Delay5/1 -> Add2/1
  z2/1 -> Delay8/1
  z1/1 -> Delay7/1
  Real-Imag to Complex/1 -> z/1
  Delay6/1 -> Add2/2
  Delay3/1 -> Add1/2
  Delay2/1 -> Add1/1
  Product4/1 -> Delay6/1
  Product3/1 -> Delay5/1
  Product1/1 -> Delay3/1
  Product/1 -> Delay2/1
  Complex to Real-Imag1/1 -> Product3/1, Product/1
  Complex to Real-Imag2/1 -> Product4/1, Product/2
  Complex to Real-Imag1/2 -> Product4/2, Product1/1
  Complex to Real-Imag2/2 -> Product3/2, Product1/2
  Add1/1 -> Delay1/1
  Add2/1 -> Delay4/1

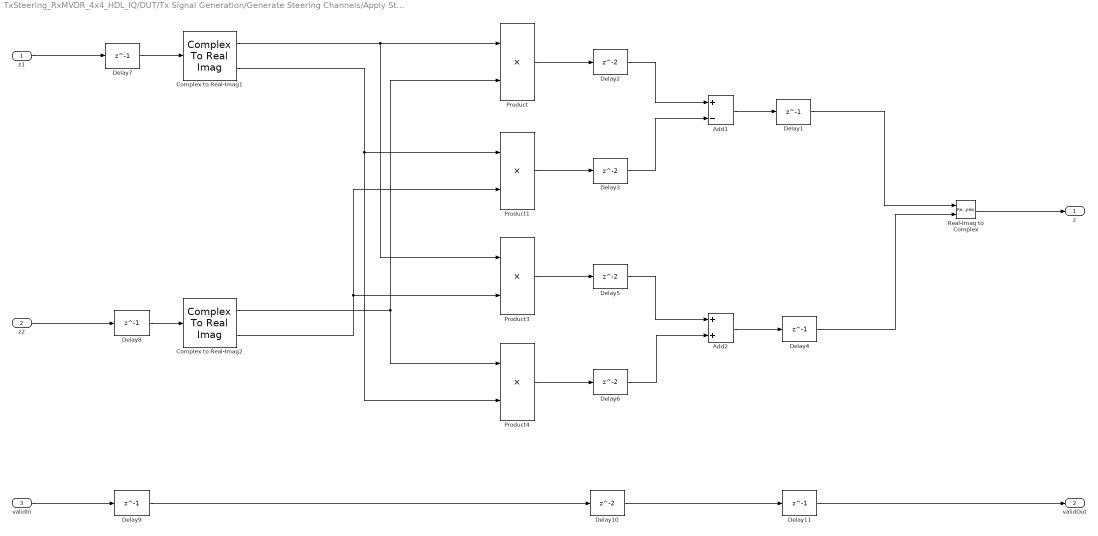
== system TxSteering_RxMVDR_4x4_HDL_IQ/DUT/Tx Signal Generation/Generate Steering Channels/Apply Steering Coefficients/HDL Complex Multiplier ==
  z1 : Inport
  z2 : Inport  Port=2
  validIn : Inport  Port=3
  Add1 : Sum  Inputs=+-
  Add2 : Sum
  Complex to Real-Imag1 : ComplexToRealImag
  Complex to Real-Imag2 : ComplexToRealImag
  Delay{1,4,7..9,11} (6 alike) : Delay  DelayLength=1  InitialCondition=0  InputProcessing=Columns as channels (frame based)
  Delay{2..3,5..6,10} (5 alike) : Delay  InitialCondition=0  InputProcessing=Columns as channels (frame based)
  Product{,1,3..4} (4 alike) : Product
  Real-Imag to Complex : RealImagToComplex
  z : Outport  VectorParamsAs1DForOutWhenUnconnected=off
  validOut : Outport  Port=2  VectorParamsAs1DForOutWhenUnconnected=off
  wires:
  Add2/1 -> Delay4/1
  Add1/1 -> Delay1/1
  Complex to Real-Imag2/2 -> Product1/2, Product3/2
  Complex to Real-Imag1/2 -> Product1/1, Product4/2
  Complex to Real-Imag2/1 -> Product/2, Product4/1
  Complex to Real-Imag1/1 -> Product/1, Product3/1
  Product/1 -> Delay2/1
  Product1/1 -> Delay3/1
  Product3/1 -> Delay5/1
  Product4/1 -> Delay6/1
  Delay2/1 -> Add1/1
  Delay3/1 -> Add1/2
  Delay6/1 -> Add2/2
  Real-Imag to Complex/1 -> z/1
  z1/1 -> Delay7/1
  z2/1 -> Delay8/1
  Delay5/1 -> Add2/1
  Delay1/1 -> Real-Imag to Complex/1
  Delay4/1 -> Real-Imag to Complex/2
  Delay7/1 -> Complex to Real-Imag1/1
  Delay8/1 -> Complex to Real-Imag2/1
  validIn/1 -> Delay9/1
  Delay9/1 -> Delay10/1
  Delay10/1 -> Delay11/1
  Delay11/1 -> validOut/1

== system TxSteering_RxMVDR_4x4_HDL_IQ/DUT/Rx Beamforming/MVDR/Compute Weight Vector/Serialize Input Data/Output Selector ==
  idx : Inport
  first : Inport  Port=2
  dataIn : Inport  Port=3
  Multiport Switch : MultiPortSwitch  DataPortOrder=Zero-based contiguous  Inputs=4  zeroidx=on
  Row 1 : Selector  NumberOfDimensions=2  InputPortWidth=3  IndexOptions=Index vector (dialog),Select all  Indices=1,1  OutputSizes=1,1
  Row 2 : Selector  NumberOfDimensions=2  InputPortWidth=3  IndexOptions=Index vector (dialog),Select all  Indices=2,1  OutputSizes=1,1
  Row 3 : Selector  NumberOfDimensions=2  InputPortWidth=3  IndexOptions=Index vector (dialog),Select all  Indices=3,1  OutputSizes=1,1
  Row 4 : Selector  NumberOfDimensions=2  InputPortWidth=3  IndexOptions=Index vector (dialog),Select all  Indices=4,1  OutputSizes=1,1
  Unit Delay Enabled Synchronous : hdlsllib/Discrete/Unit Delay Enabled Synchronous  InitialCondition=0.0  SampleTime=-1
      settings: SourceProductBaseCode=SL
  dataOut : Outport
  wires:
  Row 1/1 -> Multiport Switch/2
  Row 4/1 -> Multiport Switch/5
  Unit Delay Enabled Synchronous/1 -> Row 4/1, Row 3/1, Row 2/1
  dataIn/1 -> Unit Delay Enabled Synchronous/1, Row 1/1
  Row 2/1 -> Multiport Switch/3
  idx/1 -> Multiport Switch/1
  Row 3/1 -> Multiport Switch/4
  Multiport Switch/1 -> dataOut/1
  first/1 -> Unit Delay Enabled Synchronous/2

== system TxSteering_RxMVDR_4x4_HDL_IQ/DUT/Rx Beamforming/MVDR/Compute Weight Vector/Serialize Input Data/Output Selector1 ==
  idx : Inport
  first : Inport  Port=2
  dataIn : Inport  Port=3
  Multiport Switch : MultiPortSwitch  DataPortOrder=Zero-based contiguous  Inputs=4  zeroidx=on
  Row 1 : Selector  NumberOfDimensions=2  InputPortWidth=3  IndexOptions=Index vector (dialog),Select all  Indices=1,1  OutputSizes=1,1
  Row 2 : Selector  NumberOfDimensions=2  InputPortWidth=3  IndexOptions=Index vector (dialog),Select all  Indices=2,1  OutputSizes=1,1
  Row 3 : Selector  NumberOfDimensions=2  InputPortWidth=3  IndexOptions=Index vector (dialog),Select all  Indices=3,1  OutputSizes=1,1
  Row 4 : Selector  NumberOfDimensions=2  InputPortWidth=3  IndexOptions=Index vector (dialog),Select all  Indices=4,1  OutputSizes=1,1
  Unit Delay Enabled Synchronous : hdlsllib/Discrete/Unit Delay Enabled Synchronous  InitialCondition=0.0  SampleTime=-1
      settings: SourceProductBaseCode=SL
  dataOut : Outport
  wires:
  first/1 -> Unit Delay Enabled Synchronous/2
  Multiport Switch/1 -> dataOut/1
  Row 3/1 -> Multiport Switch/4
  idx/1 -> Multiport Switch/1
  Row 2/1 -> Multiport Switch/3
  dataIn/1 -> Row 1/1, Unit Delay Enabled Synchronous/1
  Unit Delay Enabled Synchronous/1 -> Row 2/1, Row 3/1, Row 4/1
  Row 4/1 -> Multiport Switch/5
  Row 1/1 -> Multiport Switch/2

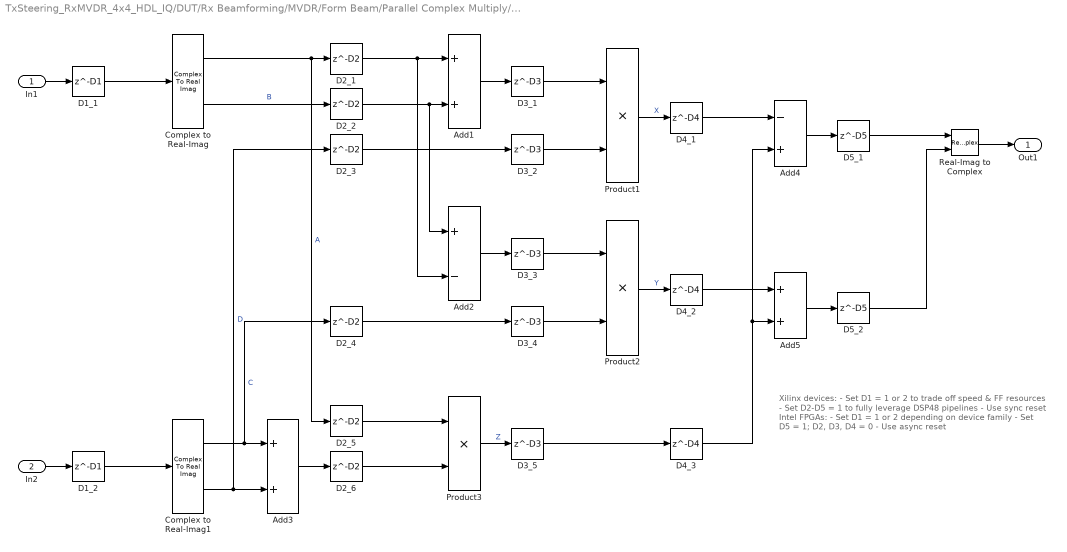
== system TxSteering_RxMVDR_4x4_HDL_IQ/DUT/Rx Beamforming/MVDR/Form Beam/Parallel Complex Multiply/HDL Complex Multiply ==
  note: Xilinx devices:
      | - Set D1 = 1 or 2 to trade off speed & FF resources
      | - Set D2-D5 = 1 to fully leverage DSP48 pipelines
      | - Use sync reset
      |
      | Intel FPGAs:
      | - Set D1 = 1 or 2 depending on device family
      | - Set D5 = 1; D2, D3, D4 = 0
      | - Use async reset
  In1 : Inport
  In2 : Inport  Port=2
  Add1 : Sum
  Add2 : Sum  Inputs=+-
  Add3 : Sum
  Add4 : Sum  Inputs=-+
  Add5 : Sum
  Complex to Real-Imag : ComplexToRealImag
  Complex to Real-Imag1 : ComplexToRealImag
  D1_1 : Delay  DelayLength=D1
  D1_2 : Delay  DelayLength=D1
  D2_{1..6} (6 alike) : Delay  DelayLength=D2
  D3_{1..5} (5 alike) : Delay  DelayLength=D3
  D4_1 : Delay  DelayLength=D4
  D4_2 : Delay  DelayLength=D4
  D4_3 : Delay  DelayLength=D4
  D5_1 : Delay  DelayLength=D5
  D5_2 : Delay  DelayLength=D5
  Product1 : Product
  Product2 : Product
  Product3 : Product
  Real-Imag to Complex : RealImagToComplex
  Out1 : Outport  VectorParamsAs1DForOutWhenUnconnected=off
  wires:
  Real-Imag to Complex/1 -> Out1/1
  In2/1 -> D1_2/1
  Complex to Real-Imag1/1 -> Add3/1, D2_4/1  "C"
  Complex to Real-Imag1/2 -> Add3/2, D2_3/1  "D"
  Product1/1 -> D4_1/1  "X"
  Product2/1 -> D4_2/1  "Y"
  Product3/1 -> D3_5/1  "Z"
  Add4/1 -> D5_1/1
  Add5/1 -> D5_2/1
  D5_1/1 -> Real-Imag to Complex/1
  D5_2/1 -> Real-Imag to Complex/2
  D4_1/1 -> Add4/1
  D4_2/1 -> Add5/1
  D3_5/1 -> D4_3/1
  Add1/1 -> D3_1/1
  Add3/1 -> D2_6/1
  Add2/1 -> D3_3/1
  Complex to Real-Imag/1 -> D2_5/1, D2_1/1  "A"
  Complex to Real-Imag/2 -> D2_2/1  "B"
  D3_1/1 -> Product1/1
  D2_6/1 -> Product3/2
  D3_3/1 -> Product2/1
  D4_3/1 -> Add4/2, Add5/2
  D3_4/1 -> Product2/2
  D3_2/1 -> Product1/2
  D2_4/1 -> D3_4/1
  D2_3/1 -> D3_2/1
  D2_5/1 -> Product3/1
  D2_2/1 -> Add1/2, Add2/1
  D2_1/1 -> Add2/2, Add1/1
  In1/1 -> D1_1/1
  D1_1/1 -> Complex to Real-Imag/1
  D1_2/1 -> Complex to Real-Imag1/1

== system TxSteering_RxMVDR_4x4_HDL_IQ/DUT/Rx Beamforming/MVDR/Form Covariance Matrix/Matrix Multiply Partitioned/Partition x_conj ==
  x : Inport
  x_conj : Inport  Port=2  Partition=on  PartitionDimension=1  PartitionWidth=1  PartitionOffset=0
  For Each : ForEach  DisableCoverage=on
  Partition x : Subsystem  TreatAsAtomicUnit=on
  C : Outport  ConcatenationDimension=1
  wires:
  x_conj/1 -> Partition x/2(x_conj_elem)
  x/1 -> Partition x/1(x)
  Partition x/1(C_col) -> C/1

== system TxSteering_RxMVDR_4x4_HDL_IQ/DUT/Rx Beamforming/MVDR/Normalize Response/MVDR Weight Update/Inner Product ==
  u : Inport
  v : Inport  Port=2
  validIn : Inport  Port=3
  Conjugate : Math  Operator=conj  SignedPower=on  RndMeth=Zero  SaturateOnIntegerOverflow=on
  Delay : Delay  DelayLength=1
  Delay1 : Delay  DelayLength=6
  Delay2 : Delay  DelayLength=ceil(log2(numArrayElements))
  Delay4 : Delay  DelayLength=1
  Element-wise complex product : Subsystem  TreatAsAtomicUnit=on
  Tree Sum with Distributed Pipelining : Subsystem
  y : Outport
  validOut : Outport  Port=2
  wires:
  v/1 -> Conjugate/1
  u/1 -> Element-wise complex product/2(v)
  validIn/1 -> Delay1/1
  Element-wise complex product/1(y) -> Delay/1
  Delay2/1 -> validOut/1
  Delay1/1 -> Delay4/1
  Delay4/1 -> Delay2/1
  Conjugate/1 -> Element-wise complex product/1(u)
  Delay/1 -> Tree Sum with Distributed Pipelining/1(In1)
  Tree Sum with Distributed Pipelining/1(Out1) -> y/1

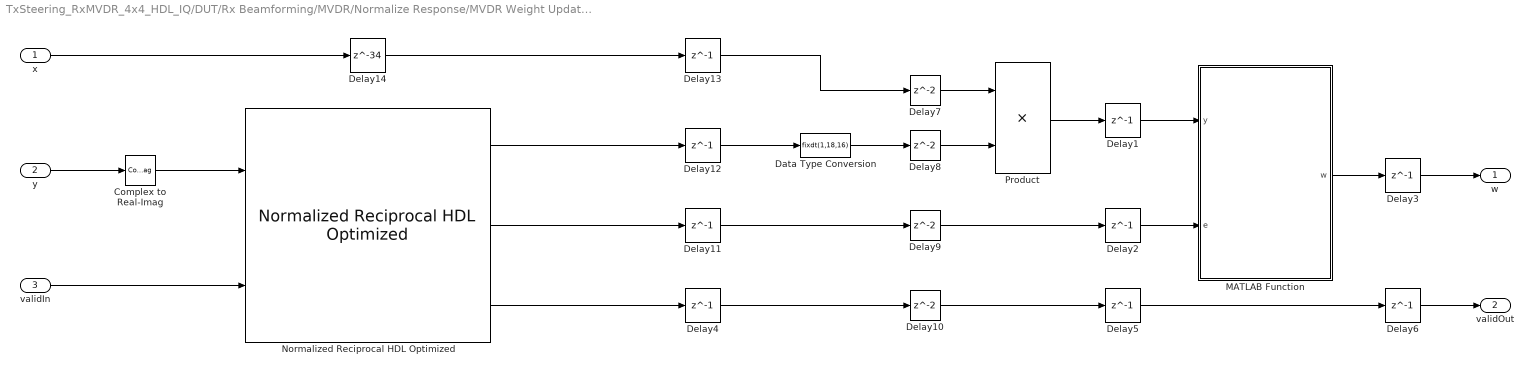
== system TxSteering_RxMVDR_4x4_HDL_IQ/DUT/Rx Beamforming/MVDR/Normalize Response/MVDR Weight Update/Vector // Scalar Divide ==
  x : Inport
  y : Inport  Port=2
  validIn : Inport  Port=3
  Complex to Real-Imag : ComplexToRealImag  Output=Real
  Data Type Conversion : DataTypeConversion  OutDataTypeStr=fixdt(1,18,16)
  Delay{1..6,11..13} (9 alike) : Delay  DelayLength=1
  Delay{7..10} (4 alike) : Delay
  Delay14 : Delay  DelayLength=34
  MATLAB Function : MATLAB Function  TreatAsAtomicUnit=on
  Normalized Reciprocal HDL Optimized : embreciprocals/Normalized Reciprocal HDL Optimized
      settings: SourceProductBaseCode=SL
  Product : Product  OutDataTypeStr=Inherit: Same as first input
  w : Outport
  validOut : Outport  Port=2
  wires:
  Delay2/1 -> MATLAB Function/2(e)
  y/1 -> Complex to Real-Imag/1
  Delay12/1 -> Data Type Conversion/1
  Complex to Real-Imag/1 -> Normalized Reciprocal HDL Optimized/1
  Delay13/1 -> Delay7/1
  Normalized Reciprocal HDL Optimized/2 -> Delay11/1
  Normalized Reciprocal HDL Optimized/1 -> Delay12/1
  Delay1/1 -> MATLAB Function/1(y)
  validIn/1 -> Normalized Reciprocal HDL Optimized/2
  Product/1 -> Delay1/1
  Delay11/1 -> Delay9/1
  MATLAB Function/1(w) -> Delay3/1
  Normalized Reciprocal HDL Optimized/3 -> Delay4/1
  Delay3/1 -> w/1
  Delay4/1 -> Delay10/1
  Delay5/1 -> Delay6/1
  Delay6/1 -> validOut/1
  x/1 -> Delay14/1
  Data Type Conversion/1 -> Delay8/1
  Delay7/1 -> Product/1
  Delay8/1 -> Product/2
  Delay9/1 -> Delay2/1
  Delay10/1 -> Delay5/1
  Delay14/1 -> Delay13/1

== system TxSteering_RxMVDR_4x4_HDL_IQ/DUT/Rx Beamforming/MVDR/Form Covariance Matrix/Matrix Multiply Partitioned/Partition x_conj/Partition x ==
  x : Inport  Partition=on  PartitionDimension=1  PartitionWidth=1  PartitionOffset=0
  x_conj_elem : Inport  Port=2
  For Each : ForEach  DisableCoverage=on
  HDL Complex Multiply : Subsystem  mask(HDL Complex Multiplier (3 Multiply, 5 Add)){D1=2, D2=1, D3=1, D4=1, D5=1}
      mask help:
      | Xilinx devices:
      | - Set D1 = 1 or 2 to trade off speed & FF resources
      | - Set D2-D5 = 1 to fully leverage DSP48 pipelines
      | - Use sync reset
      |
      | Intel FPGAs:
      | - Set D1 = 1 or 2 depending on device family
      | - Set D5 = 1; D2, D3, D4 = 0
      | - Use async reset
      mask init:
      | delay = D1+D2+D3+D4+D5;
      mask Display:
      | fprintf('Delay=%d',delay);
      | port_label('input',1,'z1');
      | port_label('input',2,'z2');
  C_col : Outport  ConcatenationDimension=1
  wires:
  x/1 -> HDL Complex Multiply/1(In1)
  x_conj_elem/1 -> HDL Complex Multiply/2(In2)
  HDL Complex Multiply/1(Out1) -> C_col/1
